simulink model "task3"  (R2023b)
settings: Solver=FixedStepDiscrete  StartTime=0.0  StopTime=20  FixedStep=5e-5  RelTol=1e-3
PreLoadFcn:
  | Simulink.defineIntEnumType('windowCommand', {'Off','Speed1','Speed2','Speed3'},[0,1,2,3])
libraries: slpidlib x2, simulink x1
settings Model: Creator=kz1nz0  LastModifiedBy=wojte

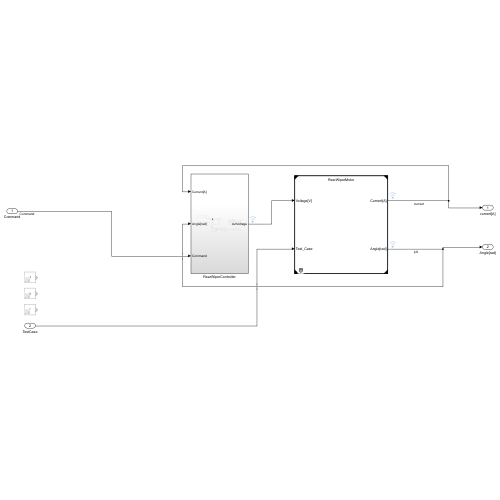
[thumbnail: Simulink's stored preview of the top-level diagram]
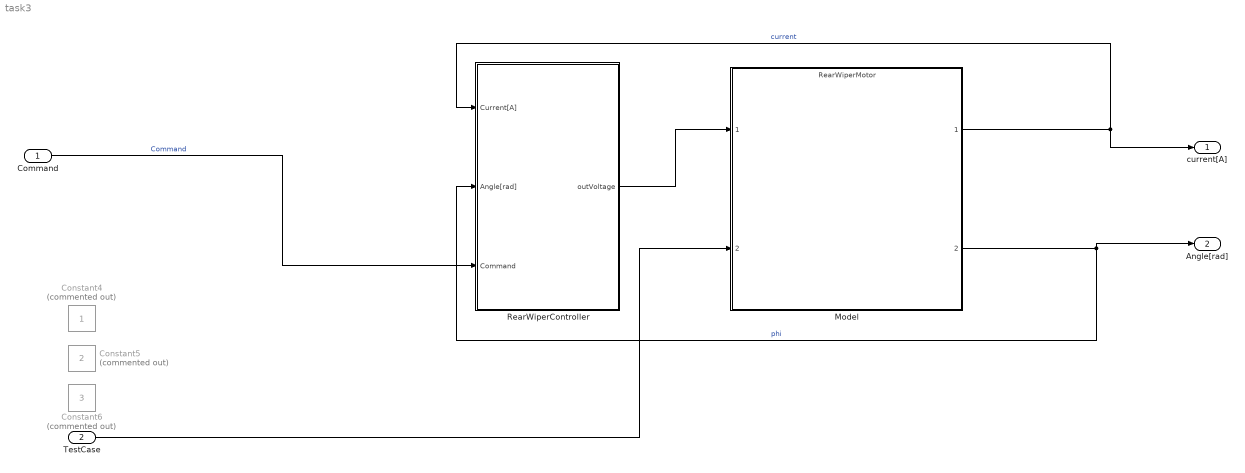
== system task3 ==
  Command : Inport  OutDataTypeStr=Enum: windowCommand
  TestCase : Inport  Port=2  OutDataTypeStr=int8
  Constant4 : Constant  Commented=on  OutDataTypeStr=int8
  Constant5 : Constant  Commented=on  Value=2  OutDataTypeStr=int8
  Constant6 : Constant  Commented=on  Value=3  OutDataTypeStr=int8
  Model : ModelReference  ModelNameDialog=RearWiperMotor.slxp  ModelReferenceVersion=19.15  CopyOfModelProtected=on
  RearWiperController : Subsystem
  current[A] : Outport
  Angle[rad] : Outport  Port=2
  wires:
  Command/1 -> RearWiperController/3(Command)  "Command"
  TestCase/1 -> Model/2
  Model/1 -> RearWiperController/1(Current[A]), current[A]/1  "current"
  Model/2 -> Angle[rad]/1, RearWiperController/2(Angle[rad])  "phi"
  RearWiperController/1(outVoltage) -> Model/1

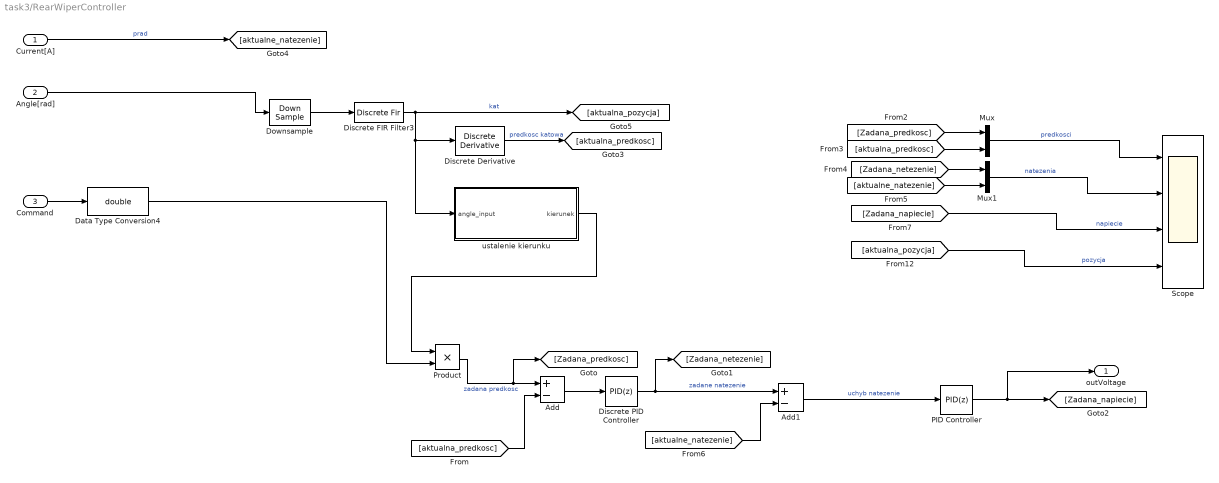
== system task3/RearWiperController ==
  Current[A] : Inport
  Angle[rad] : Inport  Port=2
  Command : Inport  Port=3
  Add : Sum  Inputs=+-
  Add1 : Sum  Inputs=+-
  Data Type Conversion4 : DataTypeConversion  OutDataTypeStr=double  SaturateOnIntegerOverflow=off  RndMeth=Floor
  Discrete Derivative : simulink/Discrete/Discrete Derivative  gainval=1.0  ICPrevScaledInput=0.0  OutMin=[]  OutMax=[]  OutDataType=fixdt(1, 16)  OutScaling=2^-10  DoSatur=off
  Discrete FIR Filter3 : DiscreteFir  Coefficients=[0.1 0.1 0.1 0.1 0.1 0.1 0.1 0.1 0.1 0.1]
  Discrete PID Controller : slpidlib/PID Controller  Controller=PID  Form=Parallel  TimeDomain=Discrete-time  UseExternalTs=off  SampleTime=-1  IntegratorMethod=Forward Euler  FilterMethod=Forward Euler  ControllerParametersSource=internal  P=9  I=40  UseKiTs=off  D=0  N=100  UseFilter=on  TunerSelectOption=Transfer Function Based (PID Tuner App)  InitialConditionSource=internal  InitialConditionForIntegrator=0  InitialConditionForFilter=0  DifferentiatorICPrevScaledInput=0  ExternalReset=none  TrackingMode=off  Kt=1  LimitOutput=on  SatLimitsSource=internal  UpperSaturationLimit=12  LowerSaturationLimit=-12  LinearizeAsGain=on  AntiWindupMode=none  Kb=1  LimitIntegrator=off  UpperIntegratorSaturationLimit=inf  LowerIntegratorSaturationLimit=-inf  POutMin=[]  POutMax=[]  IOutMin=[]  IOutMax=[]  DOutMin=[]  DOutMax=[]  NOutMin=[]  NOutMax=[]  SumOutMin=[]  SumOutMax=[]  SaturationOutMin=[]  SaturationOutMax=[]  PParamMin=[]  PParamMax=[]  IParamMin=[]  IParamMax=[]  DParamMin=[]  DParamMax=[]  NParamMin=[]  NParamMax=[]  KbParamMin=[]  KbParamMax=[]  KtParamMin=[]  KtParamMax=[]  KbOutMin=[]  KbOutMax=[]  KtOutMin=[]  KtOutMax=[]  IntegratorOutMin=[]  IntegratorOutMax=[]  FilterOutMin=[]  FilterOutMax=[]  SumI1OutMin=[]  SumI1OutMax=[]  SumI2OutMin=[]  SumI2OutMax=[]  SumI3OutMin=[]  SumI3OutMax=[]  SumI4OutMin=[]  SumI4OutMax=[]  SumDOutMin=[]  SumDOutMax=[]  DifferentiatorOutMin=[]  DifferentiatorOutMax=[]  FilterDiffOutCoefMin=[]  FilterDiffOutCoefMax=[]  ReciprocalOutMin=[]  ReciprocalOutMax=[]  SumDenOutMin=[]  SumDenOutMax=[]  SumNumOutMin=[]  SumNumOutMax=[]  DivideOutMin=[]  DivideOutMax=[]  UdiffTsProdOutMin=[]  UdiffTsProdOutMax=[]  NTsProdOutMin=[]  NTsProdOutMax=[]  UintegralTsProdOutMin=[]  UintegralTsProdOutMax=[]  UngainTsProdOutMin=[]  UngainTsProdOutMax=[]  ClampingZeroOutDataTypeStr=Inherit: Inherit via back propagation  ClampingZeroOutMin=[]  ClampingZeroOutMax=[]  FilterDenConstantOutDataTypeStr=Inherit: Inherit via back propagation  FilterDenConstantOutMin=[]  FilterDenConstantOutMax=[]  PCopyOutDataTypeStr=Inherit: Inherit via back propagation  PCopyOutMin=[]  PCopyOutMax=[]  NCopyOutDataTypeStr=Inherit: Inherit via back propagation  NCopyOutMin=[]  NCopyOutMax=[]  IntegratorContinuousStateAttributes=''  IntegratorStateMustResolveToSignalObject=off  IntegratorRTWStateStorageClass=Auto  FilterContinuousStateAttributes=''  FilterStateMustResolveToSignalObject=off  FilterRTWStateStorageClass=Auto  ParallelPVariant=InternalParameters  IdealPVariant=Disabled  IVariant=InternalParameters  DVariant=InternalParameters  IntegratorVariant=Discrete  SatVariant=Enabled  AWVariant=Passthrough  PCopyVariant=Disabled  TRVariant=Disabled  FdbkBlocksVariant=Forward  IdealPFdbkVariant=Disabled  SatFdbkVariant=Disabled  DerivativeFilterVariant=ForwardEulerFilter  NVariant=InternalParameters  NCopyVariant=Disabled  FilterICVariant=InternalICsFilter  IntegratorICVariant=InternalICs  ExternalResetVariant=Disabled  TRSumVariant=Passthrough  SumFdbkVariant=Disabled  SumVariant=Sum_PID  TsampFilterVariant=InternalTs  TsampNgainVariant=Passthrough  TsampIntegralVariant=Disabled_SignalSpec  ExternalSaturationOutDataTypeStr=Inherit: Same as second input
      settings: LibrarySourceBlock=simulink/Discrete/Discrete PID Controller
  Downsample : DownSample  N=100  RateOptions=Allow multirate processing
  Mux : Mux  Inputs=2
  Mux1 : Mux  Inputs=2
  PID Controller : slpidlib/PID Controller  Controller=PID  Form=Parallel  TimeDomain=Discrete-time  UseExternalTs=off  SampleTime=-1  IntegratorMethod=Forward Euler  FilterMethod=Forward Euler  ControllerParametersSource=internal  P=10  I=14  UseKiTs=off  D=0  N=100  UseFilter=on  TunerSelectOption=Transfer Function Based (PID Tuner App)  InitialConditionSource=internal  InitialConditionForIntegrator=0  InitialConditionForFilter=0  DifferentiatorICPrevScaledInput=0  ExternalReset=none  TrackingMode=off  Kt=1  LimitOutput=on  SatLimitsSource=internal  UpperSaturationLimit=12  LowerSaturationLimit=-12  LinearizeAsGain=on  AntiWindupMode=back-calculation  Kb=1  LimitIntegrator=off  UpperIntegratorSaturationLimit=inf  LowerIntegratorSaturationLimit=-inf  POutMin=[]  POutMax=[]  IOutMin=[]  IOutMax=[]  DOutMin=[]  DOutMax=[]  NOutMin=[]  NOutMax=[]  SumOutMin=[]  SumOutMax=[]  SaturationOutMin=[]  SaturationOutMax=[]  PParamMin=[]  PParamMax=[]  IParamMin=[]  IParamMax=[]  DParamMin=[]  DParamMax=[]  NParamMin=[]  NParamMax=[]  KbParamMin=[]  KbParamMax=[]  KtParamMin=[]  KtParamMax=[]  KbOutMin=[]  KbOutMax=[]  KtOutMin=[]  KtOutMax=[]  IntegratorOutMin=[]  IntegratorOutMax=[]  FilterOutMin=[]  FilterOutMax=[]  SumI1OutMin=[]  SumI1OutMax=[]  SumI2OutMin=[]  SumI2OutMax=[]  SumI3OutMin=[]  SumI3OutMax=[]  SumI4OutMin=[]  SumI4OutMax=[]  SumDOutMin=[]  SumDOutMax=[]  DifferentiatorOutMin=[]  DifferentiatorOutMax=[]  FilterDiffOutCoefMin=[]  FilterDiffOutCoefMax=[]  ReciprocalOutMin=[]  ReciprocalOutMax=[]  SumDenOutMin=[]  SumDenOutMax=[]  SumNumOutMin=[]  SumNumOutMax=[]  DivideOutMin=[]  DivideOutMax=[]  UdiffTsProdOutMin=[]  UdiffTsProdOutMax=[]  NTsProdOutMin=[]  NTsProdOutMax=[]  UintegralTsProdOutMin=[]  UintegralTsProdOutMax=[]  UngainTsProdOutMin=[]  UngainTsProdOutMax=[]  ClampingZeroOutDataTypeStr=Inherit: Inherit via back propagation  ClampingZeroOutMin=[]  ClampingZeroOutMax=[]  FilterDenConstantOutDataTypeStr=Inherit: Inherit via back propagation  FilterDenConstantOutMin=[]  FilterDenConstantOutMax=[]  PCopyOutDataTypeStr=Inherit: Inherit via back propagation  PCopyOutMin=[]  PCopyOutMax=[]  NCopyOutDataTypeStr=Inherit: Inherit via back propagation  NCopyOutMin=[]  NCopyOutMax=[]  IntegratorContinuousStateAttributes=''  IntegratorStateMustResolveToSignalObject=off  IntegratorRTWStateStorageClass=Auto  FilterContinuousStateAttributes=''  FilterStateMustResolveToSignalObject=off  FilterRTWStateStorageClass=Auto  ParallelPVariant=InternalParameters  IdealPVariant=Disabled  IVariant=InternalParameters  DVariant=InternalParameters  IntegratorVariant=Discrete  SatVariant=Enabled  AWVariant=BackCalculation  PCopyVariant=Disabled  TRVariant=Disabled  FdbkBlocksVariant=Forward  IdealPFdbkVariant=Disabled  SatFdbkVariant=Disabled  DerivativeFilterVariant=ForwardEulerFilter  NVariant=InternalParameters  NCopyVariant=Disabled  FilterICVariant=InternalICsFilter  IntegratorICVariant=InternalICs  ExternalResetVariant=Disabled  TRSumVariant=Passthrough  SumFdbkVariant=Disabled  SumVariant=Sum_PID  TsampFilterVariant=InternalTs  TsampNgainVariant=Passthrough  TsampIntegralVariant=Disabled_SignalSpec  ExternalSaturationOutDataTypeStr=Inherit: Same as second input
  Product : Product
  Scope : Scope  NumInputPorts=4
  ustalenie kierunku : MATLAB Function  TreatAsAtomicUnit=on
  outVoltage : Outport
  wires:
  Current[A]/1 -> [aktualne_natezenie]  "prad"
  Angle[rad]/1 -> Downsample/1
  ustalenie kierunku/1(kierunek) -> Product/1
  Discrete Derivative/1 -> [aktualna_predkosc]  "predkosc katowa"
  Downsample/1 -> Discrete FIR Filter3/1
  Product/1 -> [Zadana_predkosc], Add/1  "zadana predkosc"
  Discrete FIR Filter3/1 -> [aktualna_pozycja], ustalenie kierunku/1(angle_input), Discrete Derivative/1  "kat"
  Discrete PID Controller/1 -> Add1/1, [Zadana_netezenie]  "zadane natezenie"
  Add1/1 -> PID Controller/1  "uchyb natezenie"
  Mux/1 -> Scope/1  "predkosci"
  Mux1/1 -> Scope/2  "natezenia"
  [Zadana_predkosc] -> Mux/1
  [aktualna_predkosc] -> Mux/2
  [Zadana_netezenie] -> Mux1/1
  [aktualne_natezenie] -> Mux1/2
  [aktualne_natezenie] -> Add1/2
  [Zadana_napiecie] -> Scope/3  "napiecie"
  PID Controller/1 -> outVoltage/1, [Zadana_napiecie]
  [aktualna_pozycja] -> Scope/4  "pozycja"
  Add/1 -> Discrete PID Controller/1
  [aktualna_predkosc] -> Add/2
  Command/1 -> Data Type Conversion4/1
  Data Type Conversion4/1 -> Product/2

== matlab function task3/RearWiperController/ustalenie kierunku ==
  data: angle_input input; kierunek output
function kierunek  = fcn(angle_input)
persistent jeszcze_nie_dojechalo poprzedni_kierunek;

if isempty(jeszcze_nie_dojechalo)
    jeszcze_nie_dojechalo = true;
    poprzedni_kierunek = 1;
end

if jeszcze_nie_dojechalo
    kierunek = 1;
    if angle_input > 1
        jeszcze_nie_dojechalo = false;
    end

else %juz dojechalo 
    if angle_input >= 2.5
        kierunek = -1;
    elseif angle_input <= 0.5
        kierunek = 1;
    else
        kierunek = poprzedni_kierunek;
    end
     poprzedni_kierunek = kierunek; 
end
